simulink model "simulationUI"  (R2021a)
settings: Solver=FixedStepAuto  StartTime=0.0  StopTime=+inf  FixedStep=0.01  RelTol=1e-3
InitFcn:
  | run('system_setup.m');
undefined symbols (not defined in the file): ChargingCurrentRequest, DrivingCurrentRqst, OpenCircuitInjection, ShortCircuitInjection, sigbuilder_block, SystemState, SystemState_t
settings Model: Creator=Carlo Edoardo  LastModifiedBy=Carlo Edoardo

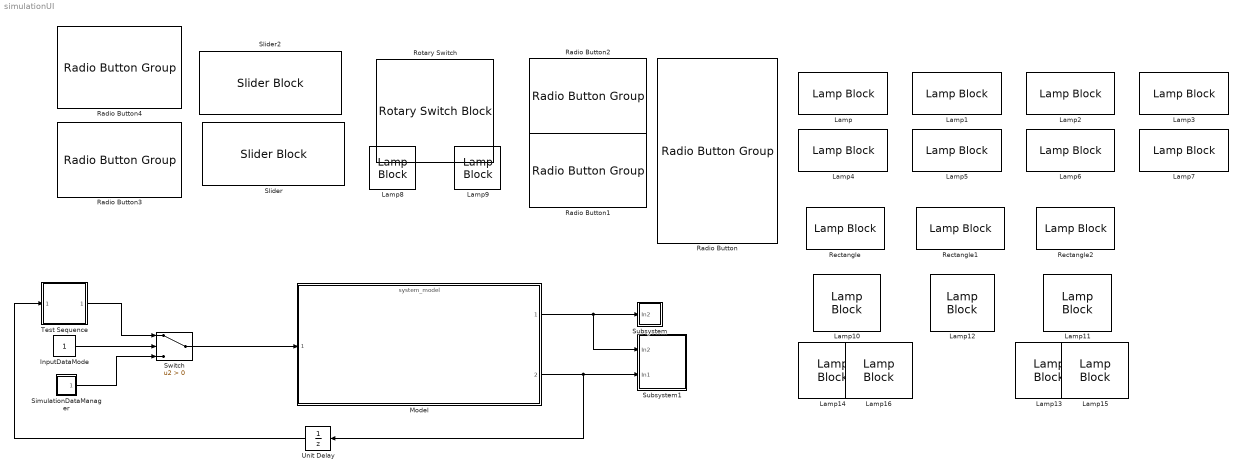
== system simulationUI ==
  InputDataMode : Constant
  Lamp{,1..7} (8 alike) : LampBlock
  Lamp{8..12} (5 alike) : LampBlock  Icon=Circle
  Lamp{13..16} (4 alike) : LampBlock  Icon=Rectangle
  Model : ModelReference  ModelNameDialog=system_model.slx  SimulationMode=Normal  ModelReferenceVersion=1.14
      mask Display: image('$imagefile'); % Use "Edit Image" on toolstrip to change.
  Radio Button : RadioButtonGroup  SelectedLabel=Cell1  ButtonGroupName=Cell
      settings: Values={{'Cell1', 'Cell2', 'Cell3', 'Cell4', 'Cell5', 'Cell6', 'Cell7', 'Cell8', 'Cell9', 'Cell10'}, [1 2 3 4 5 6 7 8 9 10]}
  Radio Button1 : RadioButtonGroup  SelectedLabel=Segment1  ButtonGroupName=Segment
      settings: Values={{'Segment1', 'Segment2', 'Segment3'}, [1 2 3]}
  Radio Button2 : RadioButtonGroup  SelectedLabel=NoFault  ButtonGroupName=FaultType
      settings: Values={{'NoFault', 'ShortCircuit', 'OpenCircuit'}, [0 1 2]}
  Radio Button3 : RadioButtonGroup  SelectedLabel=Manual  ButtonGroupName=Group
      settings: Values={{'Manual', 'FTP50'}, [1 2]}
  Radio Button4 : RadioButtonGroup  SelectedLabel=TestSequence  ButtonGroupName=Group
      settings: Values={{'Manual', 'TestSequence'}, [0 1]}
  Rectangle : LampBlock  Icon=Rectangle
  Rectangle1 : LampBlock  Icon=Rectangle
  Rectangle2 : LampBlock  Icon=Rectangle
  Rotary Switch : RotarySwitchBlock  UseEnumeratedDataType=on  EnumeratedDataType=SystemState_t
      settings: Values={{'Parking', 'Driving', 'Charging', 'Balancing'}, [0 1 2 3]}
  SimulationDataManager : Subsystem
  Slider : SliderBlock
  Slider2 : SliderBlock
  Subsystem : Subsystem
  Subsystem1 : Subsystem
  Switch : Switch  Criteria=u2 > Threshold
  Test Sequence : Test Sequence  TreatAsAtomicUnit=on
  Unit Delay : UnitDelay  SampleTime=-1  HasFrameUpgradeWarning=on
  wires:
  Model/1 -> Subsystem1/1(In2), Subsystem/1(In2)
  Model/2 -> Unit Delay/1, Subsystem1/2(In1)
  Switch/1 -> Model/1
  Test Sequence/1(BusSimulationInput) -> Switch/1
  SimulationDataManager/1(Out1) -> Switch/3
  InputDataMode/1 -> Switch/2
  Unit Delay/1 -> Test Sequence/1(BusOutputBMS)

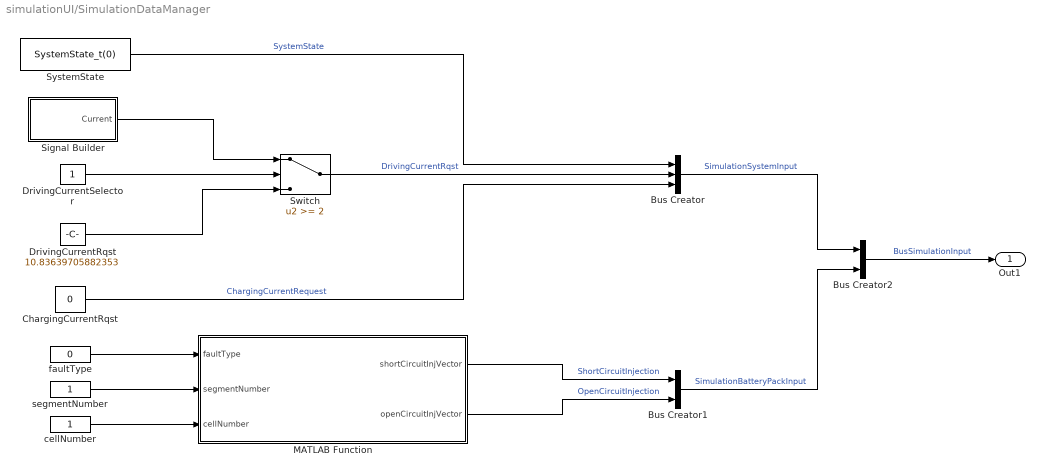
== system simulationUI/SimulationDataManager ==
  Bus Creator : BusCreator  Inputs=SystemState,DrivingCurrentRqst,ChargingCurrentRequest  OutDataTypeStr=Bus: SimulationSystemInput
  Bus Creator1 : BusCreator  Inputs=ShortCircuitInjection,OpenCircuitInjection  OutDataTypeStr=Bus: SimulationBatteryPackInput
  Bus Creator2 : BusCreator  Inputs=2  OutDataTypeStr=Bus: BusSimulationInput  NonVirtualBus=on
  ChargingCurrentRqst : Constant  Value=0
  DrivingCurrentRqst : Constant  Value=10.83639705882353
  DrivingCurrentSelector : Constant
  MATLAB Function : MATLAB Function  TreatAsAtomicUnit=on
  Signal Builder : Subsystem  Tag=STV Subsys  LoadFcn=sigbuilder_block('load');  StartFcn=sigbuilder_block('start');  StopFcn=sigbuilder_block('stop');  ClipboardFcn=sigbuilder_block('clipboard');  mask(Sigbuilder block){tuvar=[0:10]}
      mask help: Simulink:masks:SigbuilderBlock_MD
      mask init:
      | if ~strcmp(get_param(bdroot(gcbh),'SimulationStatus'),'stopped') tuvar = sigbuilder_block('maskInit'); end
      settings: CopyFcn=sigbuilder_block('copy');  DeleteFcn=sigbuilder_block('delete');  ModelCloseFcn=sigbuilder_block('modelClose');  PreSaveFcn=sigbuilder_block('preSave');  PauseFcn=sigbuilder_block('pause');  ContinueFcn=sigbuilder_block('continue');  NameChangeFcn=sigbuilder_block('namechange');  OpenFcn=sigbuilder_block('open',[1920 30 1440 722.25 ]);  CloseFcn=sigbuilder_block('close');
      mask Display: plot(0, 0, 100, 100,[2, 2, 32, 32, 2], [68, 8, 8, 68, 68],[32, 2], [38, 38], [32, 19, 2],[53, 60, 44], [32, 17, 17, 2],[16, 16, 31, 31]);txt = getActiveGroup(gcbh);text(2, 100, txt,'verticalAlignment', 'top');
  Switch : Switch  Threshold=2
  SystemState : Constant  Value=SystemState_t(0)  OutDataTypeStr=Enum: SystemState_t
  cellNumber : Constant
  faultType : Constant  Value=0
  segmentNumber : Constant
  Out1 : Outport  OutDataTypeStr=Bus: BusSimulationInput
  wires:
  Bus Creator2/1 -> Out1/1  "BusSimulationInput"
  MATLAB Function/2(openCircuitInjVector) -> Bus Creator1/2  "OpenCircuitInjection"
  segmentNumber/1 -> MATLAB Function/2(segmentNumber)
  cellNumber/1 -> MATLAB Function/3(cellNumber)
  MATLAB Function/1(shortCircuitInjVector) -> Bus Creator1/1  "ShortCircuitInjection"
  SystemState/1 -> Bus Creator/1  "SystemState"
  Bus Creator1/1 -> Bus Creator2/2  "SimulationBatteryPackInput"
  faultType/1 -> MATLAB Function/1(faultType)
  ChargingCurrentRqst/1 -> Bus Creator/3  "ChargingCurrentRequest"
  Bus Creator/1 -> Bus Creator2/1  "SimulationSystemInput"
  DrivingCurrentSelector/1 -> Switch/2
  DrivingCurrentRqst/1 -> Switch/3
  Switch/1 -> Bus Creator/2  "DrivingCurrentRqst"
  Signal Builder/1(Current) -> Switch/1

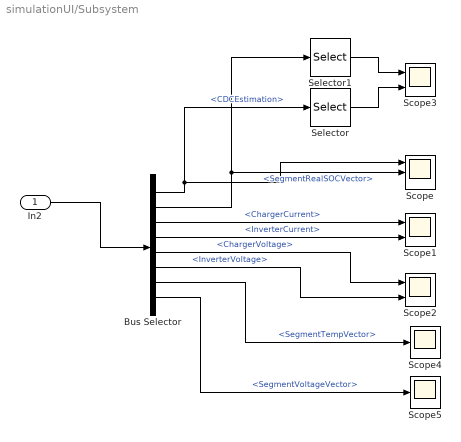
== system simulationUI/Subsystem ==
  In2 : Inport
  Bus Selector : BusSelector  OutputSignals=BusSOCEstimation.CDCEstimation,BMSBatteryPackData.SegmentRealSOCVector,SimulationChargerData.ChargerCurrent,SimulationInverterData.InverterCurrent,SimulationChargerData.ChargerVoltage,SimulationInverterData.InverterVoltage,BMSBatteryPackData.SegmentTempVector,BMSBatteryPackData.SegmentVoltageVector
  Scope : Scope  NumInputPorts=3
  Scope1 : Scope  NumInputPorts=2
  Scope2 : Scope  NumInputPorts=2
  Scope3 : Scope  NumInputPorts=2
  Scope4 : Scope
  Scope5 : Scope
  Selector : Selector  NumberOfDimensions=2  InputPortWidth=3  IndexOptions=Index vector (dialog),Index vector (dialog)  Indices=1,1  OutputSizes=1,1
  Selector1 : Selector  NumberOfDimensions=2  InputPortWidth=3  IndexOptions=Index vector (dialog),Index vector (dialog)  Indices=1,1  OutputSizes=1,1
  wires:
  Selector/1 -> Scope3/2
  Bus Selector/2 -> Selector1/1, Scope/2  "<SegmentRealSOCVector>"
  Bus Selector/3 -> Scope1/1  "<ChargerCurrent>"
  Selector1/1 -> Scope3/1
  Bus Selector/7 -> Scope4/1  "<SegmentTempVector>"
  Bus Selector/8 -> Scope5/1  "<SegmentVoltageVector>"
  Bus Selector/1 -> Selector/1, Scope/1  "<CDCEstimation>"
  Bus Selector/4 -> Scope1/2  "<InverterCurrent>"
  Bus Selector/5 -> Scope2/1  "<ChargerVoltage>"
  Bus Selector/6 -> Scope2/2  "<InverterVoltage>"
  In2/1 -> Bus Selector/1

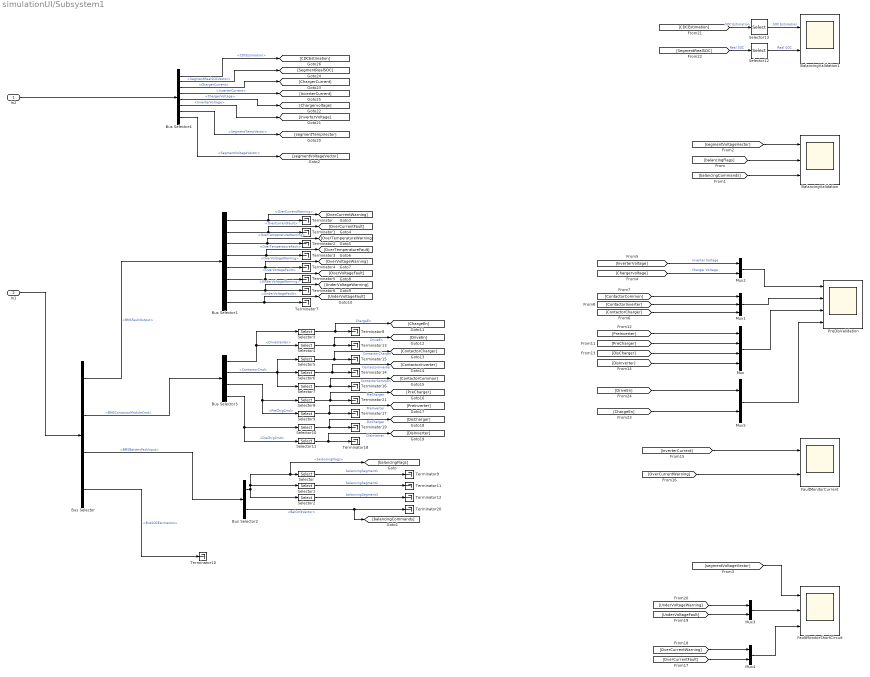
== system simulationUI/Subsystem1 ==
  In2 : Inport
  In1 : Inport  Port=2
  BalancingValidation : Scope  NumInputPorts=3
  BalancingValidation1 : Scope  NumInputPorts=2
  Bus Selector : BusSelector  OutputSignals=BMSFaultOutput,BMSContactorModuleCmd,BMSBatteryPackInput,BusSOCEstimation
  Bus Selector1 : BusSelector  OutputSignals=OverCurrentWarning,OverCurrentFault,OverTemperatureWarning,OverTemperatureFault,OverVoltageWarning,OverVoltageFault,UnderVoltageWarning,UnderVoltageFault
  Bus Selector2 : BusSelector  OutputSignals=balancingFlags,BalCmdVector
  Bus Selector3 : BusSelector  OutputSignals=DrivetrainEn,ContactorCmd,PreChrgCmd,DisChrgCmd
  Bus Selector4 : BusSelector  OutputSignals=BusSOCEstimation.CDCEstimation,BMSBatteryPackData.SegmentRealSOCVector,SimulationChargerData.ChargerCurrent,SimulationInverterData.InverterCurrent,SimulationChargerData.ChargerVoltage,SimulationInverterData.InverterVoltage,BMSBatteryPackData.SegmentTempVector,BMSBatteryPackData.SegmentVoltageVector
  FaultMonitorCurrent : Scope  NumInputPorts=2
  FaultMonitorShortCircuit : Scope  NumInputPorts=3
  Mux : Mux
  Mux1 : Mux  Inputs=3
  Mux{2..5} (4 alike) : Mux  Inputs=2
  PreDisValidation : Scope  NumInputPorts=4
  Selector : Selector  InputPortWidth=3  IndexOptions=Index vector (dialog)  Indices=1  OutputSizes=1
  Selector1 : Selector  InputPortWidth=3  IndexOptions=Index vector (dialog)  Indices=2  OutputSizes=1
  Selector10 : Selector  InputPortWidth=2  IndexOptions=Index vector (dialog)  Indices=1  OutputSizes=1
  Selector11 : Selector  InputPortWidth=2  IndexOptions=Index vector (dialog)  Indices=2  OutputSizes=1
  Selector12 : Selector  NumberOfDimensions=2  InputPortWidth=3  IndexOptions=Index vector (dialog),Index vector (dialog)  Indices=1,1  OutputSizes=1,1
  Selector13 : Selector  NumberOfDimensions=2  InputPortWidth=3  IndexOptions=Index vector (dialog),Index vector (dialog)  Indices=1,1  OutputSizes=1,1
  Selector2 : Selector  InputPortWidth=3  IndexOptions=Index vector (dialog)  Indices=3  OutputSizes=1
  Selector3 : Selector  InputPortWidth=2  IndexOptions=Index vector (dialog)  Indices=1  OutputSizes=1
  Selector4 : Selector  InputPortWidth=2  IndexOptions=Index vector (dialog)  Indices=2  OutputSizes=1
  Selector5 : Selector  InputPortWidth=3  IndexOptions=Index vector (dialog)  Indices=1  OutputSizes=1
  Selector6 : Selector  InputPortWidth=3  IndexOptions=Index vector (dialog)  Indices=2  OutputSizes=1
  Selector7 : Selector  InputPortWidth=3  IndexOptions=Index vector (dialog)  Indices=3  OutputSizes=1
  Selector8 : Selector  InputPortWidth=2  IndexOptions=Index vector (dialog)  Indices=1  OutputSizes=1
  Selector9 : Selector  InputPortWidth=2  IndexOptions=Index vector (dialog)  Indices=2  OutputSizes=1
  Terminator{,1..21} (22 alike) : Terminator
  wires:
  Bus Selector1/8 -> [UnderVoltageFault], Terminator7/1  "<UnderVoltageFault>"
  Bus Selector1/3 -> [OverTemperatureWarning], Terminator2/1  "<OverTemperatureWarning>"
  Bus Selector/1 -> Bus Selector1/1  "<BMSFaultOutput>"
  Bus Selector1/2 -> [OverCurrentFault], Terminator1/1  "<OverCurrentFault>"
  Bus Selector1/5 -> [OverVoltageWarning], Terminator4/1  "<OverVoltageWarning>"
  Bus Selector1/6 -> [OverVoltageFault], Terminator5/1  "<OverVoltageFault>"
  Bus Selector1/4 -> [OverTemperatureFault], Terminator3/1  "<OverTemperatureFault>"
  Bus Selector1/1 -> [OverCurrentWarning], Terminator/1  "<OverCurrentWarning>"
  Bus Selector1/7 -> [UnderVoltageWarning], Terminator6/1  "<UnderVoltageWarning>"
  Bus Selector/4 -> Terminator10/1  "<BusSOCEstimation>"
  Bus Selector/3 -> Bus Selector2/1  "<BMSBatteryPackInput>"
  Bus Selector/2 -> Bus Selector3/1  "<BMSContactorModuleCmd>"
  In1/1 -> Bus Selector/1
  Selector/1 -> Terminator9/1  "balancingSegment1"
  Selector1/1 -> Terminator11/1  "balancingSegment2"
  Selector2/1 -> Terminator12/1  "balancingSegment3"
  Bus Selector2/1 -> [balancingFlags], Selector/1, Selector1/1, Selector2/1  "<balancingFlags>"
  Bus Selector3/1 -> Selector4/1, Selector3/1  "<DrivetrainEn>"
  Selector3/1 -> [ChargeEn], Terminator8/1  "ChargeEn"
  Selector4/1 -> [DriveEn], Terminator13/1  "DriveEn"
  Selector6/1 -> [ContactorInverter], Terminator14/1  "ContactorInverter"
  Selector5/1 -> [ContactorCharger], Terminator15/1  "ContactorCharger"
  Bus Selector3/2 -> Selector7/1, Selector6/1, Selector5/1  "<ContactorCmd>"
  Selector7/1 -> [ContactorCommon], Terminator16/1  "ContactorCommon"
  Selector10/1 -> [DisCharger], Terminator19/1  "DisCharger"
  Selector11/1 -> [DisInverter], Terminator18/1  "DisInverter"
  Selector9/1 -> [PreInverter], Terminator17/1  "PreInverter"
  Selector8/1 -> [PreCharger], Terminator21/1  "PreCharger"
  Bus Selector3/3 -> Selector9/1, Selector8/1  "<PreChrgCmd>"
  Bus Selector3/4 -> Selector11/1, Selector10/1  "<DisChrgCmd>"
  Bus Selector2/2 -> [balancingCommands], Terminator20/1  "<BalCmdVector>"
  Bus Selector4/5 -> [Chargervoltage]  "<ChargerVoltage>"
  Bus Selector4/6 -> [InverterVoltage]  "<InverterVoltage>"
  Bus Selector4/3 -> [ChargerCurrent]  "<ChargerCurrent>"
  In2/1 -> Bus Selector4/1
  Bus Selector4/4 -> [InverterCurrent]  "<InverterCurrent>"
  Bus Selector4/7 -> [segmentTempVector]  "<SegmentTempVector>"
  Bus Selector4/1 -> [CDCEstimation]  "<CDCEstimation>"
  Bus Selector4/2 -> [SegmentRealSOC]  "<SegmentRealSOCVector>"
  Bus Selector4/8 -> [segmentVoltageVector]  "<SegmentVoltageVector>"
  [balancingFlags] -> BalancingValidation/2
  [balancingCommands] -> BalancingValidation/3
  [segmentVoltageVector] -> BalancingValidation/1
  [segmentVoltageVector] -> FaultMonitorShortCircuit/1
  Mux/1 -> PreDisValidation/3
  Mux1/1 -> PreDisValidation/2
  Mux2/1 -> PreDisValidation/1
  [Chargervoltage] -> Mux2/2  "Charger Voltage"
  [InverterVoltage] -> Mux2/1  "Inverter Voltage"
  [ContactorCharger] -> Mux1/3
  [ContactorCommon] -> Mux1/1
  [ContactorInverter] -> Mux1/2
  [PreCharger] -> Mux/2
  [PreInverter] -> Mux/1
  [DisCharger] -> Mux/3
  [DisInverter] -> Mux/4
  [InverterCurrent] -> FaultMonitorCurrent/1
  [OverCurrentWarning] -> FaultMonitorCurrent/2
  Mux3/1 -> FaultMonitorShortCircuit/2
  Mux4/1 -> FaultMonitorShortCircuit/3
  [OverCurrentFault] -> Mux4/2
  [OverCurrentWarning] -> Mux4/1
  [UnderVoltageFault] -> Mux3/2
  [UnderVoltageWarning] -> Mux3/1
  [CDCEstimation] -> Selector13/1  "SOC Estimation"
  [SegmentRealSOC] -> Selector12/1  "Real SOC"
  Selector13/1 -> BalancingValidation1/1  "SOC Estimation"
  Selector12/1 -> BalancingValidation1/2  "Real SOC"
  [DriveEn] -> Mux5/1
  [ChargeEn] -> Mux5/2
  Mux5/1 -> PreDisValidation/4

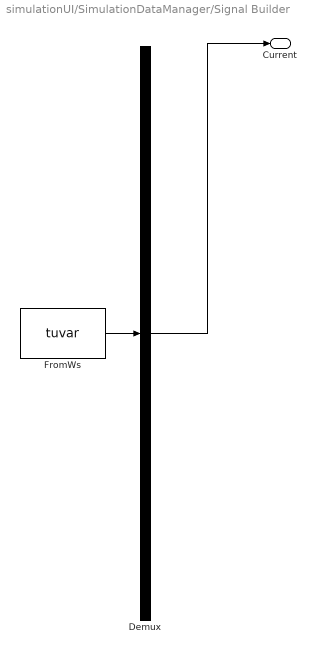
== system simulationUI/SimulationDataManager/Signal Builder ==
  Demux : Demux  Tag=STV Demux  Outputs=1
      settings: DisplayOption=none
  FromWs : FromWorkspace  Tag=STV FromWs  VariableName=tuvar
      SigBuilderData=|
      | common.afterFinalStr = 'Extrapolate'
      | common.sampleTime = 0
      | dataSet.timeRange = [0 2474]
      | dataSet.name = 'FTP-75 Drive Cycle'
      | sbobj.Groups.Name = 'FTP-75 Drive Cycle'
      | sbobj.Groups.Signals.Name = 'Current'
      | sbobj.Groups.Signals.XData = [0 0.00166966283167 0.00489865696245 0.00887290141926 0.01 0.0132228027433 0.0164456054866 0.0196684082299 0.02 0.0216579588505 0.0216579588505 0.023878217756 ... (264079 elements, 1x264079)]
      | sbobj.Groups.Signals.YData = [0 0 0 0 0 0 0 0 0 0 -7.47487403974e-31 -1.06202348499e-17 ... (264079 elements, 1x264079)]
      | sbobj.Groups.TimeRange = [0 2474]
  Current : Outport  Tag=STV Outport
  wires:
  Demux/1 -> Current/1
  FromWs/1 -> Demux/1

== matlab function simulationUI/SimulationDataManager/MATLAB Function ==
  data: faultType input; shortCircuitInjVector output; segmentNumber input; cellNumber input; openCircuitInjVector output
function [shortCircuitInjVector, openCircuitInjVector] = faultInjectionParser(faultType, segmentNumber, cellNumber)

switch(faultType)
    case 0
        shortCircuitInjVector=false(3,10);
        openCircuitInjVector=false(3,10);
    case 1
        shortCircuitInjVector=false(3,10);
        openCircuitInjVector=false(3,10);
        shortCircuitInjVector(segmentNumber, cellNumber)=true;
    case 2
        shortCircuitInjVector=false(3,10);
        openCircuitInjVector=false(3,10);
        openCircuitInjVector(segmentNumber, cellNumber)=true;
    otherwise 
        shortCircuitInjVector=false(3,10);
        openCircuitInjVector=false(3,10);
end

== stateflow chart simulationUI/Test Sequence ==
  state Init
    BusSimulationInput.SimulationSystemInput.SystemState = SystemState_t.Parking;
    BusSimulationInput.SimulationSystemInput.DrivingCurrentRqst = 0;
    BusSimulationInput.SimulationSystemInput.ChargingCurrentRequest = 0;
    BusSimulationInput.SimulationBatteryPackInput.ShortCircuitInjection = false(3,10);
    BusSimulationInput.SimulationBatteryPackInput.OpenCircuitInjection = false(3,10);
  state DrivingPrecharge
    BusSimulationInput.SimulationSystemInput.SystemState = SystemState_t.Driving;
  state Driving10A
    BusSimulationInput.SimulationSystemInput.DrivingCurrentRqst = 10;
  state Driving20A
    BusSimulationInput.SimulationSystemInput.DrivingCurrentRqst = 20;
  state Driving25A
    BusSimulationInput.SimulationSystemInput.DrivingCurrentRqst = 25;
  state Parking1
    BusSimulationInput.SimulationSystemInput.DrivingCurrentRqst = 0;
    BusSimulationInput.SimulationSystemInput.SystemState = SystemState_t.Parking;
  state ChargingPrecharge
    BusSimulationInput.SimulationSystemInput.SystemState = SystemState_t.Charging;
  state Charging2A
    BusSimulationInput.SimulationSystemInput.ChargingCurrentRequest = 2;
  state Parking2
    BusSimulationInput.SimulationSystemInput.ChargingCurrentRequest = 0;
    BusSimulationInput.SimulationSystemInput.SystemState = SystemState_t.Parking;
  state FaultInjection
    BusSimulationInput.SimulationBatteryPackInput.ShortCircuitInjection(1,1) = true;
  state RemoveFault
    BusSimulationInput.SimulationBatteryPackInput.ShortCircuitInjection = false(3,10);
  state Balancing
    BusSimulationInput.SimulationSystemInput.SystemState = SystemState_t.Balancing;
  state ParkingEnd
    BusSimulationInput.SimulationSystemInput.SystemState = SystemState_t.Parking;
    BusSimulationInput.SimulationSystemInput.DrivingCurrentRqst = 0;
    BusSimulationInput.SimulationSystemInput.ChargingCurrentRequest = 0;
    BusSimulationInput.SimulationBatteryPackInput.ShortCircuitInjection = false(3,10);
    BusSimulationInput.SimulationBatteryPackInput.OpenCircuitInjection = false(3,10);
  (default) -> Init
  Init -> DrivingPrecharge : [
      | after(500,msec)
      | ]
  DrivingPrecharge -> Driving10A : [
      | BusOutputBMS.BMSContactorModuleCmd.DrivetrainEn(2)==1
      | ]
  Driving10A -> Driving20A : [
      | after(40000, msec)
      | ]
  Driving20A -> Driving25A : [
      | after(30000,msec)
      | ]
  Driving25A -> Parking1 : [
      | after(20000,msec)
      | ]
  Parking1 -> ChargingPrecharge : [
      | BusOutputBMS.BMSContactorModuleCmd.DrivetrainEn(2)==0&& BusOutputBMS.BMSContactorModuleCmd.DisChrgCmd(2)== 0
      | ]
  ChargingPrecharge -> Charging2A : [
      | BusOutputBMS.BMSContactorModuleCmd.DrivetrainEn(1)== 1
      | ]
  Charging2A -> Parking2 : [
      | after(5000,msec)
      | ]
  Parking2 -> FaultInjection : [
      | BusOutputBMS.BMSContactorModuleCmd.DrivetrainEn(1)==0 && BusOutputBMS.BMSContactorModuleCmd.DisChrgCmd(1)== 0
      | ]
  FaultInjection -> RemoveFault : [
      | after(200,msec)
      | ]
  RemoveFault -> Balancing
  Balancing -> ParkingEnd : [
      | BusOutputBMS.BMSBatteryPackInput.balancingFlags(1)==0 && BusOutputBMS.BMSBatteryPackInput.balancingFlags(2)==0 && BusOutputBMS.BMSBatteryPackInput.balancingFlags(3)==0
      | ]
  data: BusSimulationInput output Bus: BusSimulationInput; BusOutputBMS input Bus: BusOutputBMS
